simulink model "PositionPIDcontrol_REALTIME"  (R2020b)
settings: Solver=ode3  StartTime=0.0  StopTime=5  FixedStep=0.001  RelTol=1e-3
values from neighbouring files (symbols this model uses):
  ctrl =     [PID_params_LAB0.mat]
undefined symbols (not defined in the file or in its folder): DiscIntNeverNeededParam, National_Instruments, PCI, sens, step_size
libraries: sldrtlib x3, simulink x2
settings Model: ExtModeTrigDuration=10000  Creator=39345  LastModifiedBy=tortoranic
settings DataIOCC: ReturnWorkspaceOutputs=off
settings RTWCC: Description=Simulink Desktop Real-Time  SystemTargetFile=sldrt.tlc  TemplateMakefile=sldrt.tmf  RTWCompilerOptimization=on
settings CodeAppCC: MaxIdLength=95
settings SimulinkDesktopRealTimeCC: TargetPreCompLibLocation=C:\Program Files\MATLAB\R2020b\toolbox\sldrt\lib\win64

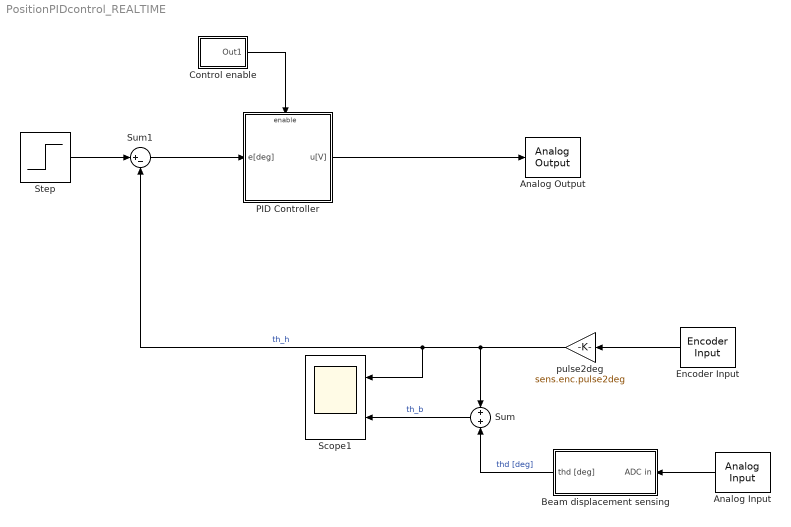
== system PositionPIDcontrol_REALTIME ==
  Analog Input : sldrtlib/Analog Input  SampleTime=0.001  MaxMissedTicks=10  ShowMissedTicks=off  YieldWhenWaiting=off  DrvName=National_Instruments/PCI-6221  DrvAddress=4294967295  DrvOptions=[0 0 0 2 0]  Channels=[3 4]  RangeMode=1  VoltRange=2  DataType=1
      settings: AttributesFormatString=National Instruments\nPCI-6221 [auto]
  Analog Output : sldrtlib/Analog Output  SampleTime=0.001  MaxMissedTicks=10  ShowMissedTicks=off  YieldWhenWaiting=off  DrvName=National_Instruments/PCI-6221  DrvAddress=4294967295  DrvOptions=[0 0 0 2 0]  Channels=1  RangeMode=1  VoltRange=1  InitialValue=0  FinalValue=0
      settings: AttributesFormatString=National Instruments\nPCI-6221 [auto]
  Beam displacement sensing : Subsystem
  Control enable : Subsystem
  Encoder Input : sldrtlib/Encoder Input  SampleTime=0.001  MaxMissedTicks=10  ShowMissedTicks=off  YieldWhenWaiting=off  DrvName=National_Instruments/PCI-6221  DrvAddress=4294967295  DrvOptions=[0 0 0 2 0]  Channels=1  QuadMode=3  IndexPulse=1  InputFilter=Inf  DataType=1
      settings: AttributesFormatString=National Instruments\nPCI-6221 [auto]
  PID Controller : Subsystem
  Scope1 : Scope  NumInputPorts=2
  Step : Step  After=step_size  SampleTime=0.001
  Sum : Sum
  Sum1 : Sum  Inputs=|+-
  pulse2deg : Gain  Gain=sens.enc.pulse2deg
  wires:
  Sum/1 -> Scope1/2  "th_b"
  Encoder Input/1 -> pulse2deg/1
  pulse2deg/1 -> Scope1/1, Sum1/2, Sum/1  "th_h"
  Step/1 -> Sum1/1
  Sum1/1 -> PID Controller/1(e[deg])
  PID Controller/1(u[V]) -> Analog Output/1
  Analog Input/1 -> Beam displacement sensing/1(ADC in)
  Beam displacement sensing/1(thd [deg]) -> Sum/2  "thd [deg]"
  Control enable/1(Out1) -> PID Controller/Enable

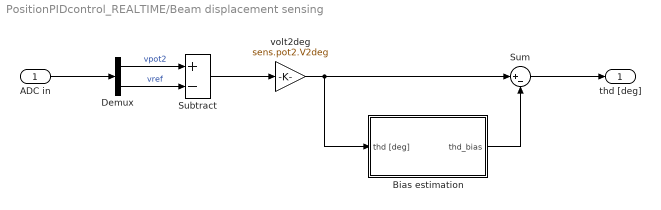
== system PositionPIDcontrol_REALTIME/Beam displacement sensing ==
  ADC in : Inport
  Bias estimation : Subsystem
  Demux : Demux  Outputs=2
  Subtract : Sum  Inputs=+-
  Sum : Sum  Inputs=|+-
  volt2deg : Gain  Gain=sens.pot2.V2deg
  thd [deg] : Outport
  wires:
  Subtract/1 -> volt2deg/1
  Demux/1 -> Subtract/1  "vpot2"
  Demux/2 -> Subtract/2  "vref"
  ADC in/1 -> Demux/1
  volt2deg/1 -> Bias estimation/1(thd [deg]), Sum/1
  Bias estimation/1(thd_bias) -> Sum/2
  Sum/1 -> thd [deg]/1

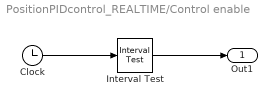
== system PositionPIDcontrol_REALTIME/Control enable ==
  Clock : Clock
  Interval Test : simulink/Logic and Bit Operations/Interval Test  IntervalClosedRight=on  uplimit=60  IntervalClosedLeft=on  lowlimit=0.7  OutDataTypeStr=boolean
  Out1 : Outport
  wires:
  Clock/1 -> Interval Test/1
  Interval Test/1 -> Out1/1

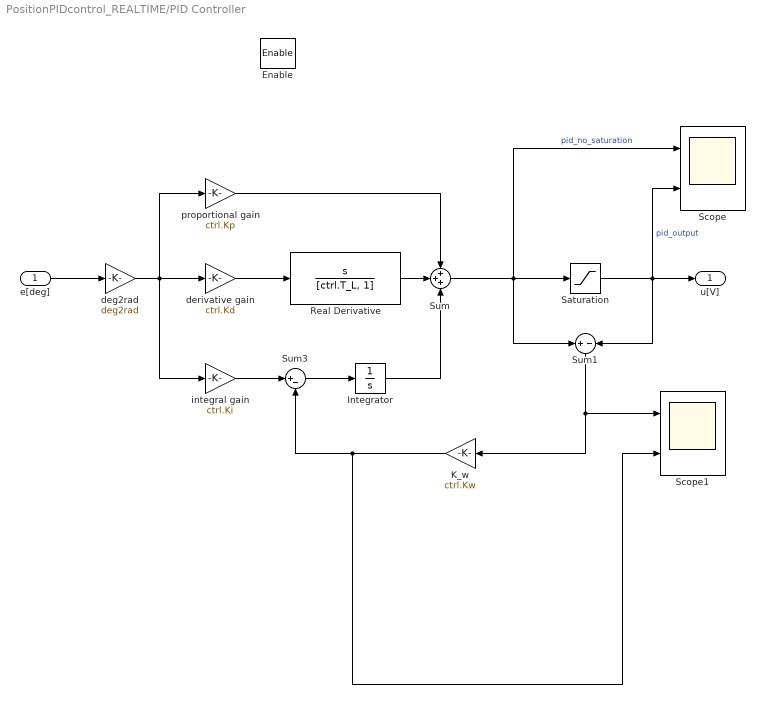
== system PositionPIDcontrol_REALTIME/PID Controller ==
  e[deg] : Inport
  Enable : EnablePort  StatesWhenEnabling=reset
  Integrator : Integrator
  K_w : Gain  Gain=ctrl.Kw
  Real Derivative : TransferFcn  Numerator=[1 0]  Denominator=[ctrl.T_L, 1]
  Saturation : Saturate  UpperLimit=10  LowerLimit=-10
  Scope : Scope  NumInputPorts=2
  Scope1 : Scope  NumInputPorts=2
  Sum : Sum  Inputs=+++
  Sum1 : Sum  Inputs=+|-
  Sum3 : Sum  Inputs=|+-
  deg2rad : Gain  Gain=deg2rad
  derivative gain : Gain  Gain=ctrl.Kd
  integral gain : Gain  Gain=ctrl.Ki
  proportional gain : Gain  Gain=ctrl.Kp
  u[V] : Outport
  wires:
  Real Derivative/1 -> Sum/2
  proportional gain/1 -> Sum/1
  Sum1/1 -> Scope1/1, K_w/1
  derivative gain/1 -> Real Derivative/1
  deg2rad/1 -> integral gain/1, derivative gain/1, proportional gain/1
  Integrator/1 -> Sum/3
  integral gain/1 -> Sum3/1
  Sum3/1 -> Integrator/1
  K_w/1 -> Scope1/2, Sum3/2
  e[deg]/1 -> deg2rad/1
  Sum/1 -> Scope/1, Saturation/1, Sum1/1  "pid_no_saturation"
  Saturation/1 -> Scope/2, u[V]/1, Sum1/2  "pid_output"

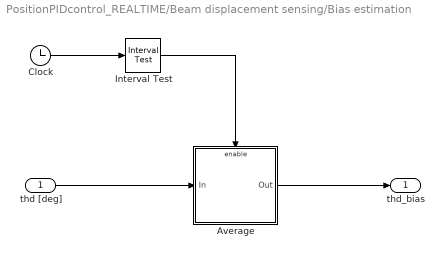
== system PositionPIDcontrol_REALTIME/Beam displacement sensing/Bias estimation ==
  thd [deg] : Inport
  Average : Subsystem
  Clock : Clock
  Interval Test : simulink/Logic and Bit Operations/Interval Test  IntervalClosedRight=on  uplimit=0.7  IntervalClosedLeft=on  lowlimit=0.2  OutDataTypeStr=boolean
  thd_bias : Outport
  wires:
  Clock/1 -> Interval Test/1
  thd [deg]/1 -> Average/1(In)
  Average/1(Out) -> thd_bias/1
  Interval Test/1 -> Average/Enable

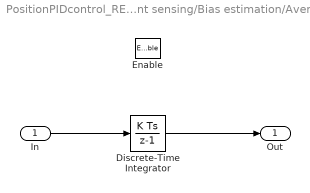
== system PositionPIDcontrol_REALTIME/Beam displacement sensing/Bias estimation/Average ==
  In : Inport
  Enable : EnablePort
  Discrete-Time Integrator : DiscreteIntegrator  gainval=2.0  SampleTime=0.001  ICPrevOutput=DiscIntNeverNeededParam  ICPrevScaledInput=DiscIntNeverNeededParam
  Out : Outport
  wires:
  In/1 -> Discrete-Time Integrator/1
  Discrete-Time Integrator/1 -> Out/1
